simulink model "ControleFF_trajetoria_D_integrado"  (R2020a)
settings: Solver=ode23  StartTime=0.0  StopTime=60  FixedStep=rate  RelTol=1e-3
values from neighbouring files (symbols this model uses):
  Beff = 50    [Ex4.m]    (also in initializeRobotParameters.m; plot_angular_positions.m; plot_angular_positions_RRR.m; testeIntegracao.m)
  Jeff = 2.2    [Ex4.m]    (also in initializeRobotParameters.m = 0.5; plot_angular_positions.m = 0.5; plot_angular_positions_RRR.m = 0.5; testeIntegracao.m = 0.5)
  K = 17.7    [Ex4.m]    (also in initializeRobotParameters.m = 0.785398163397; plot_angular_positions.m = 0.785398163397; plot_angular_positions_RRR.m = 0.785398163397; testeIntegracao.m = 0.785398163397)
  Kd = (2*qsi*wn*Jeff - Beff)/K    (= -0.338983050847)    [Ex4.m]    (also in initializeRobotParameters.m = -44.5633840657; plot_angular_positions.m = -44.5633840657; plot_angular_positions_RRR.m = -44.5633840657; testeIntegracao.m = -44.5633840657)
  Kp = (wn^2*Jeff)/K    (= 12.4293785311)    [Ex4.m]    (also in initializeRobotParameters.m = 143.239448783; plot_angular_positions.m = 143.239448783; plot_angular_positions_RRR.m = 143.239448783; testeIntegracao.m = 143.239448783)
  N = 10    [Ex4.m]    (also in initializeRobotParameters.m = 3; plot_angular_positions.m = 3; plot_angular_positions_RRR.m = 3; testeIntegracao.m = 3)
  r = 0.01    [Ex4.m]    (also in initializeRobotParameters.m = 1./[231.22*4 139.138 139.138 231.22 231.22]; plot_angular_positions.m = 1./[231.22*4 139.138 139.138 231.22 231.22]; plot_angular_positions_RRR.m = 1./[231.22*4 139.138 139.138]; testeIntegracao.m = 1./[231.22*4 139.138 139.138 231.22 231.22])
  SP_theta = [0, 0, 0]    [Ex4.m]    (also in SP_theta.mat = [1.57079632679 0.0274016692563 0 0 0]; testeIntegracao.m = [0 0 0 0 0]; testes.m = [0,0,0,0,0])
libraries: simulink_extras x6
(part 5 of 5)

== matlab function ControleFF_trajetoria_D_integrado/Compensador Feedforward/Perturbação_d/MATLAB Function3 ==
  data: M input; V input; tau1 output; G input; ddTh input
function tau1  = calcul_dk1(M, V, G, ddTh)

tau1 = M(1,2)*ddTh(2) + M(1,3)*ddTh(3) + M(1,4)*ddTh(4) + M(1,5)*ddTh(5) ...
       + V(1) + G(1);
